simulink model "mbed_disco_f429_SerialLoop"  (R2015a)
settings: Solver=FixedStepDiscrete  SolverMode=SingleTasking  StartTime=0.0  StopTime=10.0  FixedStep=1e-3  RelTol=1e-3
libraries: mbed_lib x2, mbed_targets_stm_disco_f429 x1
settings Model: CovSFcnEnable=off  Creator=oh  LastModifiedBy=oh
settings OptimizationCC: OptimizeModelRefInitCode=on  LifeSpan=1
settings DebuggingCC: SolverPrmCheckMsg=warning
settings HardwareCC: ProdLargestAtomicInteger=Long  ProdLargestAtomicFloat=Double  ProdEndianess=LittleEndian  ProdHWDeviceType=ARM Compatible->ARM Cortex
settings RTWCC: SystemTargetFile=mbed.tlc  TemplateMakefile=mbed.tmf  Description=Mbed Target (Embedded Target)  TargetLang=C++
settings CodeAppCC: IgnoreCustomStorageClasses=off
settings STFCustomTargetCC: CombineOutputUpdateFcns=on  SupportContinuousTime=off  SupportVariableSizeSignals=off  SystemTargetFile=mbed.tlc
settings ERTTargetCC: SupportContinuousTime=off  SupportVariableSizeSignals=off  ERTCustomFileTemplate=mbed_file_process.tlc

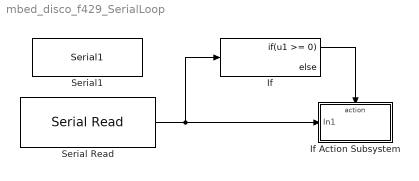
== system mbed_disco_f429_SerialLoop ==
  If : If  IfExpression=u1 >= 0
  If Action Subsystem : Subsystem  TreatAsAtomicUnit=on
  Serial Read : mbed_lib/Serial/Serial Read  SParameter1=Serial1  SampleTime=-1
  Serial1 : mbed_targets_stm_disco_f429/Serial1  Parameter1=0
  wires:
  Serial Read/1 -> If Action Subsystem/1(In1), If/1
  If/1 -> If Action Subsystem/Action

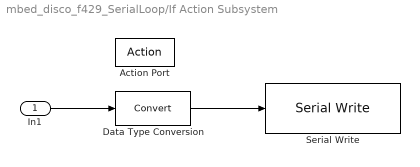
== system mbed_disco_f429_SerialLoop/If Action Subsystem ==
  In1 : Inport
  Action Port : ActionPort  ActionType=then
  Data Type Conversion : DataTypeConversion
  Serial Write : mbed_lib/Serial/Serial Write  SParameter1=Serial1  SampleTime=-1
  wires:
  Data Type Conversion/1 -> Serial Write/1
  In1/1 -> Data Type Conversion/1
